simulink model "q9"  (R2020b)
settings: Solver=VariableStepAuto  StartTime=0.0  StopTime=10.0  RelTol=1e-3
PreLoadFcn:
  | Ts=1e-5;
  | flux=0.2158;
  | trap=0.5;
  | B=7.92721e-6;
  | J=92.5/1000;
  | P=8;
  | R=0.6;
  | L=0.00028;
  | K=25.5/1000;
settings Model: Creator=Akshay A H  LastModifiedBy=Ravi

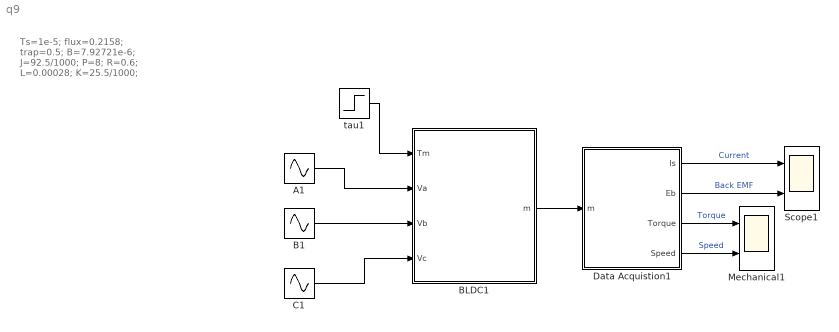
== system q9 ==
  note: Ts=1e-5;
      | flux=0.2158;
      | trap=0.5;
      | B=7.92721e-6;
      | J=92.5/1000;
      | P=8;
      | R=0.6;
      | L=0.00028;
      | K=25.5/1000;
  A1 : Sin  Amplitude=220*sqrt(2)  Frequency=2*pi*50  SampleTime=Ts
  B1 : Sin  Amplitude=220*sqrt(2)  Frequency=2*pi*50  Phase=-2*pi/3  SampleTime=Ts
  BLDC1 : Subsystem  mask(Brushless DC Motor :){Rs=1.43, Ls=9.4e-3, flux=0.2158, J=1.5e-3, B=2e-3, p=4}
      mask prompts: Rs "Resistance - Rs [ohms] :"; Ls "Inductance - Ls [H] :"; flux "Flux - [wb]"; J "Rotor Inertia - J [kg-m^2]"; B "Friction Coefficient - B :"; p "No: poles of Motor :"
      mask help: Brushless DC Motor inducing trapezoidal Back EMF
      mask init:
      | trap=0.5;
      mask Display: fprintf('BLDC')
  C1 : Sin  Amplitude=220*sqrt(2)  Frequency=2*pi*50  Phase=2*pi/3  SampleTime=Ts
  Data Acquistion1 : Subsystem
  Mechanical1 : Scope  NumInputPorts=2
  Scope1 : Scope  NumInputPorts=2
  tau1 : Step  Time=0.5  After=10  SampleTime=0
  wires:
  Data Acquistion1/4(Speed) -> Mechanical1/2  "Speed"
  B1/1 -> BLDC1/3(Vb)
  Data Acquistion1/3(Torque) -> Mechanical1/1  "Torque"
  BLDC1/1(m) -> Data Acquistion1/1(m)
  A1/1 -> BLDC1/2(Va)
  Data Acquistion1/2(Eb) -> Scope1/2  "Back EMF"
  Data Acquistion1/1(Is) -> Scope1/1  "Current"
  tau1/1 -> BLDC1/1(Tm)
  C1/1 -> BLDC1/4(Vc)

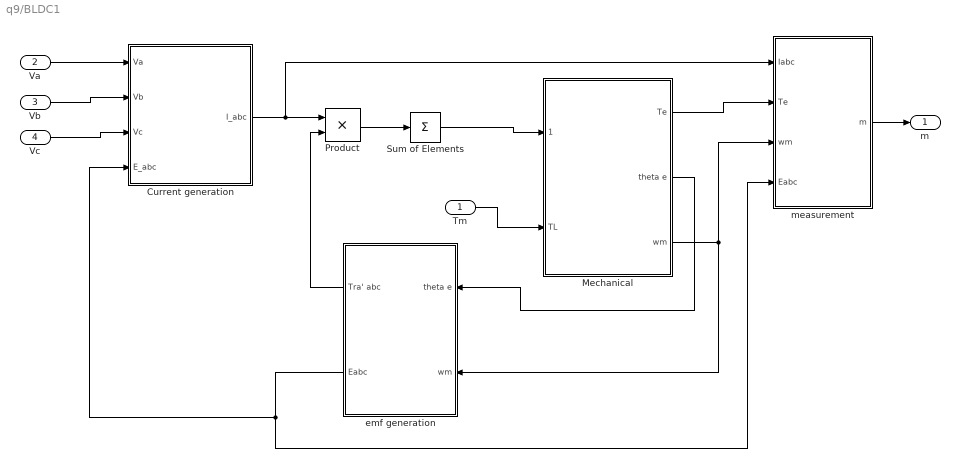
== system q9/BLDC1 ==
  Tm : Inport
  Va : Inport  Port=2
  Vb : Inport  Port=3
  Vc : Inport  Port=4
  Current generation : Subsystem
  Mechanical : Subsystem
  Product : Product  SaturateOnIntegerOverflow=on  OutDataTypeStr=Inherit: Same as first input
  Sum of Elements : Sum  Inputs=+
  emf generation : Subsystem
  measurement : Subsystem
  m : Outport
  wires:
  Vc/1 -> Current generation/3(Vc)
  Vb/1 -> Current generation/2(Vb)
  Va/1 -> Current generation/1(Va)
  measurement/1(m) -> m/1
  Mechanical/2(theta e) -> emf generation/1(theta e)
  Mechanical/3(wm) -> measurement/3(wm), emf generation/2(wm)
  Tm/1 -> Mechanical/2(TL)
  emf generation/1(Tra' abc) -> Product/2
  Product/1 -> Sum of Elements/1
  emf generation/2(Eabc) -> Current generation/4(E_abc), measurement/4(Eabc)
  Current generation/1(I_abc) -> Product/1, measurement/1(Iabc)
  Mechanical/1(Te) -> measurement/2(Te)
  Sum of Elements/1 -> Mechanical/1(1)

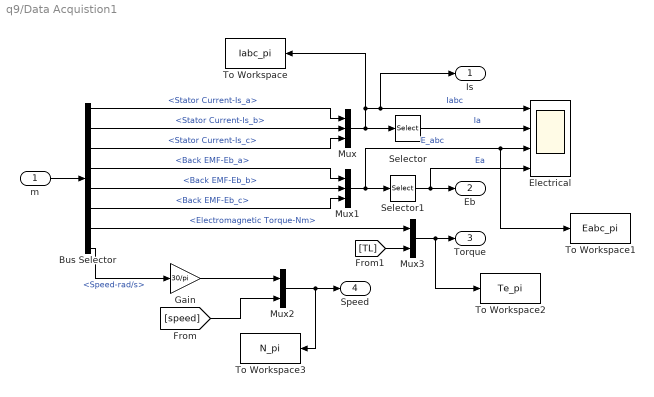
== system q9/Data Acquistion1 ==
  m : Inport
  Bus Selector : BusSelector  OutputSignals=Stator Current-Is_a,Stator Current-Is_b,Stator Current-Is_c,Back EMF-Eb_a,Back EMF-Eb_b,Back EMF-Eb_c,Electromagnetic Torque-Nm,Speed-rad/s
  Electrical : Scope  NumInputPorts=4
  Gain : Gain  Gain=30/pi
  Mux : Mux  Inputs=3
  Mux1 : Mux  Inputs=3
  Mux2 : Mux  Inputs=2
  Mux3 : Mux  Inputs=2
  Selector : Selector  InputPortWidth=3  IndexOptions=Index vector (dialog)  Indices=[1 ]  OutputSizes=1
  Selector1 : Selector  InputPortWidth=3  IndexOptions=Index vector (dialog)  Indices=[1 ]  OutputSizes=1
  To Workspace : ToWorkspace  VariableName=Iabc_pi  SampleTime=Ts
  To Workspace1 : ToWorkspace  VariableName=Eabc_pi  SampleTime=Ts
  To Workspace2 : ToWorkspace  VariableName=Te_pi  SampleTime=Ts
  To Workspace3 : ToWorkspace  VariableName=N_pi  SampleTime=Ts
  Is : Outport
  Eb : Outport  Port=2
  Torque : Outport  Port=3
  Speed : Outport  Port=4
  wires:
  Mux3/1 -> To Workspace2/1, Torque/1
  [TL] -> Mux3/2
  [speed] -> Mux2/2
  Mux2/1 -> To Workspace3/1, Speed/1
  Gain/1 -> Mux2/1
  Selector1/1 -> Electrical/4, Eb/1  "Ea"
  Selector/1 -> Electrical/2  "Ia"
  Bus Selector/8 -> Gain/1  "<Speed-rad/s>"
  Bus Selector/7 -> Mux3/1  "<Electromagnetic Torque-Nm>"
  Mux1/1 -> To Workspace1/1, Electrical/3, Selector1/1  "E_abc"
  Bus Selector/6 -> Mux1/3  "<Back EMF-Eb_c>"
  Bus Selector/5 -> Mux1/2  "<Back EMF-Eb_b>"
  Bus Selector/4 -> Mux1/1  "<Back EMF-Eb_a>"
  Mux/1 -> Is/1, Electrical/1, To Workspace/1, Selector/1  "Iabc"
  Bus Selector/3 -> Mux/3  "<Stator Current-Is_c>"
  Bus Selector/2 -> Mux/2  "<Stator Current-Is_b>"
  Bus Selector/1 -> Mux/1  "<Stator Current-Is_a>"
  m/1 -> Bus Selector/1

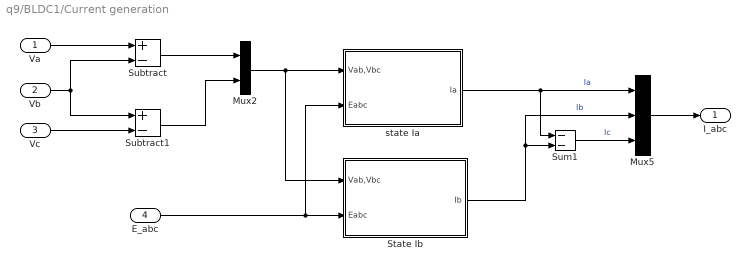
== system q9/BLDC1/Current generation ==
  Va : Inport
  Vb : Inport  Port=2
  Vc : Inport  Port=3
  E_abc : Inport  Port=4
  Mux2 : Mux  Inputs=2
  Mux5 : Mux  Inputs=3
  State Ib : Subsystem
  Subtract : Sum  Inputs=+-
  Subtract1 : Sum  Inputs=+-
  Sum1 : Sum  Inputs=--  SaturateOnIntegerOverflow=on
  state Ia : Subsystem
  I_abc : Outport
  wires:
  State Ib/1(Ib) -> Sum1/2, Mux5/2  "Ib"
  Subtract1/1 -> Mux2/2
  Subtract/1 -> Mux2/1
  Vc/1 -> Subtract1/2
  Vb/1 -> Subtract1/1, Subtract/2
  Va/1 -> Subtract/1
  state Ia/1(Ia) -> Mux5/1, Sum1/1  "Ia"
  Sum1/1 -> Mux5/3  "Ic"
  Mux5/1 -> I_abc/1
  Mux2/1 -> State Ib/1(Vab,Vbc), state Ia/1(Vab,Vbc)
  E_abc/1 -> State Ib/2(Eabc), state Ia/2(Eabc)

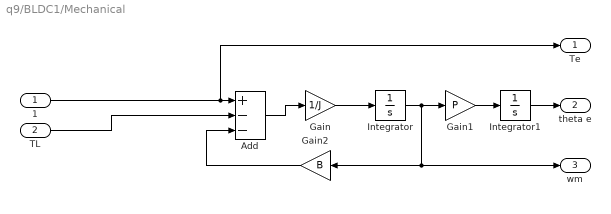
== system q9/BLDC1/Mechanical ==
  1 : Inport
  TL : Inport  Port=2
  Add : Sum  Inputs=+--
  Gain : Gain  Gain=1/J
  Gain1 : Gain  Gain=P
  Gain2 : Gain  Gain=B
  Integrator : Integrator
  Integrator1 : Integrator
  Te : Outport
  theta e : Outport  Port=2
  wm : Outport  Port=3
  wires:
  Integrator/1 -> Gain2/1, wm/1, Gain1/1
  Add/1 -> Gain/1
  Gain/1 -> Integrator/1
  Gain1/1 -> Integrator1/1
  1/1 -> Te/1, Add/1
  TL/1 -> Add/2
  Gain2/1 -> Add/3
  Integrator1/1 -> theta e/1

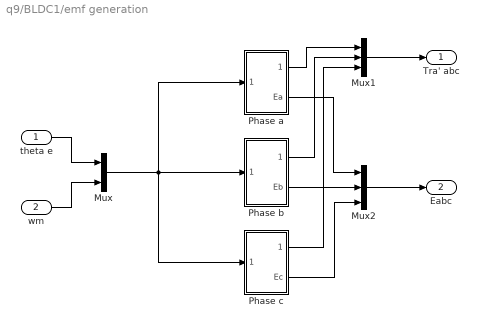
== system q9/BLDC1/emf generation ==
  theta e : Inport
  wm : Inport  Port=2
  Mux : Mux  Inputs=2
  Mux1 : Mux  Inputs=3
  Mux2 : Mux  Inputs=3
  Phase a : Subsystem
  Phase b : Subsystem
  Phase c : Subsystem
  Tra' abc : Outport
  Eabc : Outport  Port=2
  wires:
  wm/1 -> Mux/2
  theta e/1 -> Mux/1
  Mux/1 -> Phase a/1(In1), Phase c/1(In1), Phase b/1(In1)
  Phase c/2(Ec) -> Mux2/3
  Mux1/1 -> Tra' abc/1
  Phase a/1(Tra' a) -> Mux1/1
  Phase c/1(Tra' c) -> Mux1/3
  Phase b/1(Tra' b) -> Mux1/2
  Phase b/2(Eb) -> Mux2/2
  Phase a/2(Ea) -> Mux2/1
  Mux2/1 -> Eabc/1

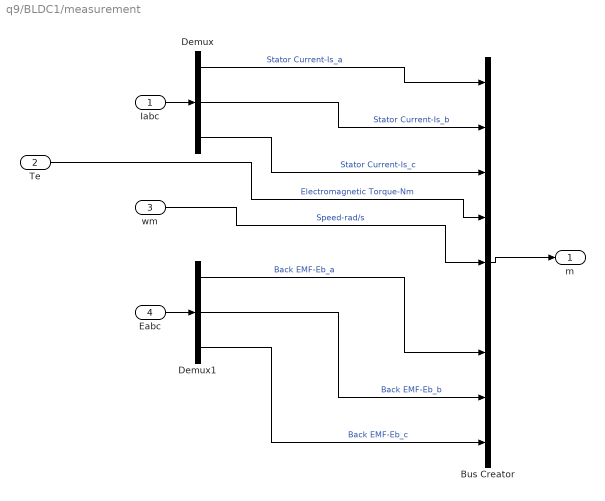
== system q9/BLDC1/measurement ==
  Iabc : Inport
  Te : Inport  Port=2
  wm : Inport  Port=3
  Eabc : Inport  Port=4
  Bus Creator : BusCreator  Inputs=9
  Demux : Demux  Outputs=3
  Demux1 : Demux  Outputs=3
  m : Outport
  wires:
  ? -> Bus Creator/6  "rotor theta-rad"
  Demux1/3 -> Bus Creator/9  "Back EMF-Eb_c"
  Demux1/2 -> Bus Creator/8  "Back EMF-Eb_b"
  Demux1/1 -> Bus Creator/7  "Back EMF-Eb_a"
  Eabc/1 -> Demux1/1
  Demux/2 -> Bus Creator/2  "Stator Current-Is_b"
  Bus Creator/1 -> m/1
  wm/1 -> Bus Creator/5  "Speed-rad/s"
  Te/1 -> Bus Creator/4  "Electromagnetic Torque-Nm"
  Demux/3 -> Bus Creator/3  "Stator Current-Is_c"
  Demux/1 -> Bus Creator/1  "Stator Current-Is_a"
  Iabc/1 -> Demux/1

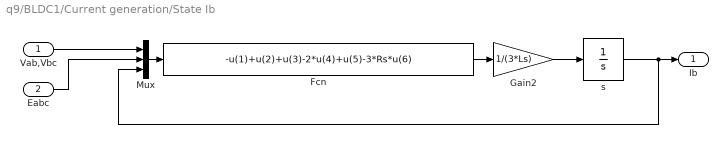
== system q9/BLDC1/Current generation/State Ib ==
  Vab,Vbc : Inport
  Eabc : Inport  Port=2
  Fcn : Fcn  Expr=-u(1)+u(2)+u(3)-2*u(4)+u(5)-3*Rs*u(6)
  Gain2 : Gain  Gain=1/(3*Ls)  SaturateOnIntegerOverflow=on  OutDataTypeStr=Inherit: Same as input  ParamDataTypeStr=Inherit: Same as input
  Mux : Mux  Inputs=3
  "s " : Integrator
  Ib : Outport
  wires:
  "s "/1 -> Ib/1, Mux/3
  Fcn/1 -> Gain2/1
  Mux/1 -> Fcn/1
  Eabc/1 -> Mux/2
  Vab,Vbc/1 -> Mux/1
  Gain2/1 -> "s "/1

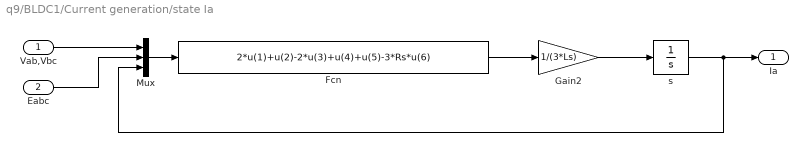
== system q9/BLDC1/Current generation/state Ia ==
  Vab,Vbc : Inport
  Eabc : Inport  Port=2
  Fcn : Fcn  Expr=2*u(1)+u(2)-2*u(3)+u(4)+u(5)-3*Rs*u(6)
  Gain2 : Gain  Gain=1/(3*Ls)  SaturateOnIntegerOverflow=on  OutDataTypeStr=Inherit: Same as input  ParamDataTypeStr=Inherit: Same as input
  Mux : Mux  Inputs=3
  "s " : Integrator
  Ia : Outport
  wires:
  Gain2/1 -> "s "/1
  Vab,Vbc/1 -> Mux/1
  Eabc/1 -> Mux/2
  Mux/1 -> Fcn/1
  Fcn/1 -> Gain2/1
  "s "/1 -> Ia/1, Mux/3

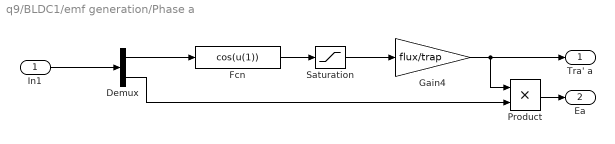
== system q9/BLDC1/emf generation/Phase a ==
  In1 : Inport
  Demux : Demux  Outputs=2
  Fcn : Fcn  Expr=cos(u(1))
  Gain4 : Gain  Gain=flux/trap  SaturateOnIntegerOverflow=on  OutDataTypeStr=Inherit: Same as input  ParamDataTypeStr=Inherit: Same as input
  Product : Product
  Saturation : Saturate  UpperLimit=trap  LowerLimit=-trap
  Tra' a : Outport
  Ea : Outport  Port=2
  wires:
  Product/1 -> Ea/1
  In1/1 -> Demux/1
  Demux/2 -> Product/2
  Demux/1 -> Fcn/1
  Gain4/1 -> Tra' a/1, Product/1
  Saturation/1 -> Gain4/1
  Fcn/1 -> Saturation/1

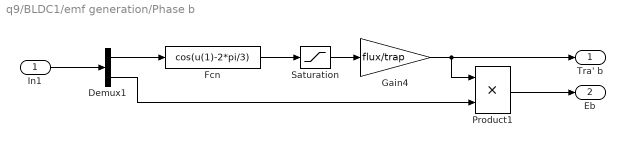
== system q9/BLDC1/emf generation/Phase b ==
  In1 : Inport
  Demux1 : Demux  Outputs=2
  Fcn : Fcn  Expr=cos(u(1)-2*pi/3)
  Gain4 : Gain  Gain=flux/trap  SaturateOnIntegerOverflow=on  OutDataTypeStr=Inherit: Same as input  ParamDataTypeStr=Inherit: Same as input
  Product1 : Product  SaturateOnIntegerOverflow=on  OutDataTypeStr=Inherit: Same as first input
  Saturation : Saturate  UpperLimit=trap  LowerLimit=-trap
  Tra' b : Outport
  Eb : Outport  Port=2
  wires:
  Demux1/1 -> Fcn/1
  Product1/1 -> Eb/1
  In1/1 -> Demux1/1
  Gain4/1 -> Tra' b/1, Product1/1
  Demux1/2 -> Product1/2
  Fcn/1 -> Saturation/1
  Saturation/1 -> Gain4/1

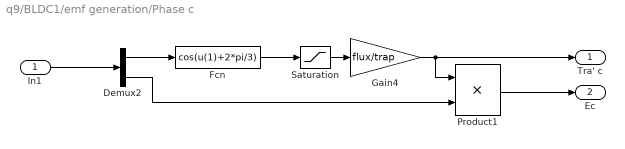
== system q9/BLDC1/emf generation/Phase c ==
  In1 : Inport
  Demux2 : Demux  Outputs=2
  Fcn : Fcn  Expr=cos(u(1)+2*pi/3)
  Gain4 : Gain  Gain=flux/trap  SaturateOnIntegerOverflow=on  OutDataTypeStr=Inherit: Same as input  ParamDataTypeStr=Inherit: Same as input
  Product1 : Product  SaturateOnIntegerOverflow=on  OutDataTypeStr=Inherit: Same as first input
  Saturation : Saturate  UpperLimit=trap  LowerLimit=-trap
  Tra' c : Outport
  Ec : Outport  Port=2
  wires:
  In1/1 -> Demux2/1
  Gain4/1 -> Tra' c/1, Product1/1
  Fcn/1 -> Saturation/1
  Demux2/2 -> Product1/2
  Saturation/1 -> Gain4/1
  Product1/1 -> Ec/1
  Demux2/1 -> Fcn/1
